simulink model "Punto_6a"  (R2022a)
settings: Solver=VariableStepAuto  StartTime=0.0  StopTime=10.0  RelTol=1e-3
undefined symbols (not defined in the file): A, alpha, B, beta
settings Model: Creator=garzo  LastModifiedBy=garzo

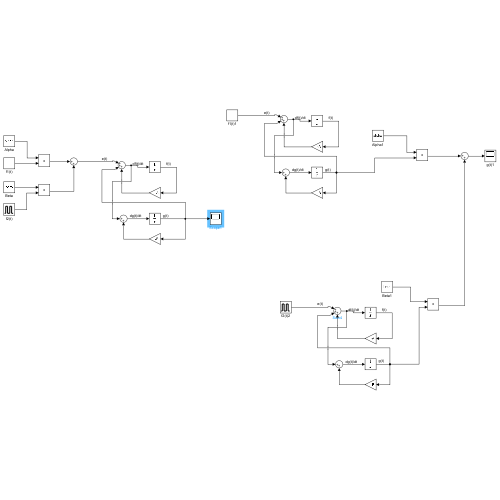
[thumbnail: Simulink's stored preview of the top-level diagram]
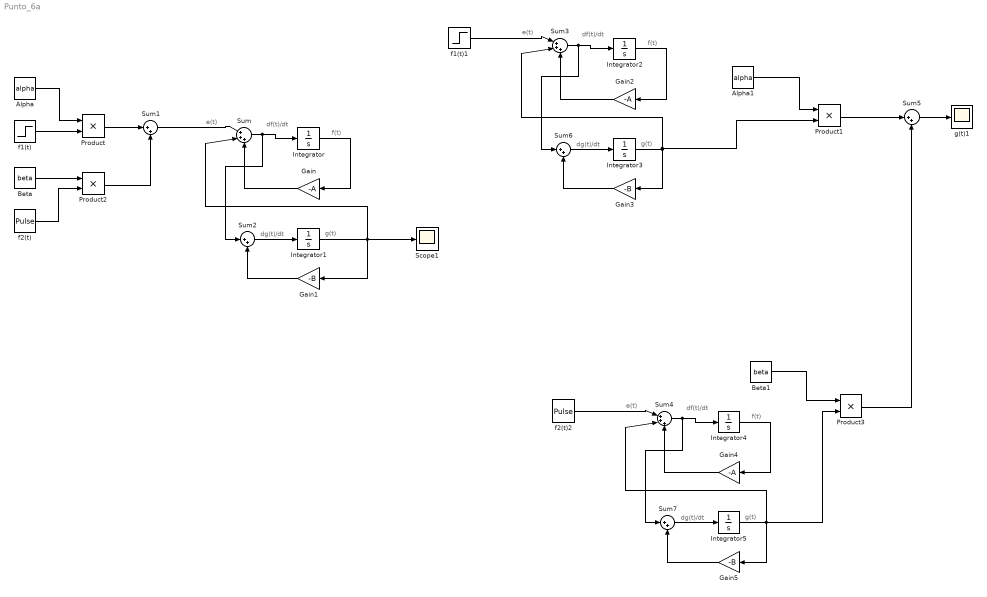
== system Punto_6a ==
  note: e(t)
  note: g(t)
  note: f(t)
  note: dg(t)/dt
  note: df(t)/dt
  note: e(t)
  note: g(t)
  note: f(t)
  note: dg(t)/dt
  note: df(t)/dt
  note: df(t)/dt
  note: e(t)
  note: dg(t)/dt
  note: f(t)
  note: g(t)
  Alpha : Constant  Value=alpha
  Alpha1 : Constant  Value=alpha
  Beta : Constant  Value=beta
  Beta1 : Constant  Value=beta
  Gain : Gain  Gain=-A
  Gain1 : Gain  Gain=-B
  Gain2 : Gain  Gain=-A
  Gain3 : Gain  Gain=-B
  Gain4 : Gain  Gain=-A
  Gain5 : Gain  Gain=-B
  Integrator{,1..5} (6 alike) : Integrator
  Product{,1..3} (4 alike) : Product
  Scope1 : Scope
  Sum : Sum  Inputs=|+++
  Sum{1..2,5..7} (5 alike) : Sum  Inputs=|++
  Sum3 : Sum  Inputs=|+++
  Sum4 : Sum  Inputs=|+++
  f1(t) : Step  SampleTime=0
  f1(t)1 : Step  SampleTime=0
  f2(t) : DiscretePulseGenerator  PulseType=Time based  Period=10  PulseWidth=5
  f2(t)2 : DiscretePulseGenerator  PulseType=Time based  Period=10  PulseWidth=5
  g(t)1 : Scope
  wires:
  Alpha/1 -> Product/1
  f1(t)/1 -> Product/2
  f2(t)/1 -> Product2/2
  Product2/1 -> Sum1/2
  Product/1 -> Sum1/1
  Beta/1 -> Product2/1
  Integrator/1 -> Gain/1
  Sum1/1 -> Sum/1
  Integrator1/1 -> Sum/2, Scope1/1, Gain1/1
  Gain1/1 -> Sum2/2
  Sum/1 -> Sum2/1, Integrator/1
  Gain/1 -> Sum/3
  Sum2/1 -> Integrator1/1
  Product1/1 -> Sum5/1
  Beta1/1 -> Product3/1
  Product3/1 -> Sum5/2
  Alpha1/1 -> Product1/1
  Sum5/1 -> g(t)1/1
  Integrator2/1 -> Gain2/1
  f1(t)1/1 -> Sum3/1
  Gain3/1 -> Sum6/2
  Sum3/1 -> Sum6/1, Integrator2/1
  Gain2/1 -> Sum3/3
  Sum6/1 -> Integrator3/1
  Integrator3/1 -> Product1/2, Sum3/2, Gain3/1
  Integrator5/1 -> Product3/2, Sum4/2, Gain5/1
  Gain4/1 -> Sum4/3
  Sum4/1 -> Sum7/1, Integrator4/1
  Integrator4/1 -> Gain4/1
  f2(t)2/1 -> Sum4/1
  Gain5/1 -> Sum7/2
  Sum7/1 -> Integrator5/1
